simulink model "five_bots_Observer_Obstacle_1_sin_cir"  (R2019b)
settings: Solver=ode5  StartTime=0.0  StopTime=35.0  FixedStep=0.005  RelTol=1e-3
(part 3 of 3)

== matlab function five_bots_Observer_Obstacle_1_sin_cir/Self Calculation 3/APF & Reference Correction/Subsystem/Abstract ==
  data: reference input; agent_x_d output; agent_dot_x_d output; agent_ddot_x_d output
function [agent_x_d, agent_dot_x_d, agent_ddot_x_d] = abstract(reference)

% This function will pick out the reference for the current agent

%% basic parameters
num_agent = 5;
serial_num = 3;
dimension = 3;

% abstract the reference position
x_d = reference (dimension*num_agent*0+1:dimension*num_agent*1);
dot_x_d = reference (dimension*num_agent*1+1:dimension*num_agent*2);
ddot_x_d = reference (dimension*num_agent*2+1:dimension*num_agent*3);

% get the reference for the current agent
agent_x_d = x_d (dimension*(serial_num-1)+1 : dimension*serial_num);
agent_dot_x_d = dot_x_d (dimension*(serial_num-1)+1 : dimension*serial_num);
agent_ddot_x_d = ddot_x_d (dimension*(serial_num-1)+1 : dimension*serial_num);

end

== matlab function five_bots_Observer_Obstacle_1_sin_cir/Self Calculation 3/APF & Reference Correction/Subsystem/Error calculation ==
  data: agent_x_d input; agent_dot_x_d input; pos input; delta_x output; vel input; delta_v output
function [delta_x, delta_v] = error_calculation(agent_x_d, agent_dot_x_d, pos, vel)

delta_x = pos - agent_x_d;
delta_v = vel - agent_dot_x_d;

end

== matlab function five_bots_Observer_Obstacle_1_sin_cir/Self Calculation 3/APF & Reference Correction/Subsystem/Reference Correction ==
  data: agent_x_d input; agent_dot_x_d input; agent_ddot_x_d input; new_x_d output; ob_info input; pos input; vel input; flag_ob input; new_dot_x_d output; new_ddot_x_d output; k_i output
function [new_x_d, new_dot_x_d, new_ddot_x_d,k_i] = fcn(agent_x_d, agent_dot_x_d, agent_ddot_x_d, ob_info, pos, vel, flag_ob)

%% Note
% This function calculates the reference tracking error according to the
% current reference

% input:
% agent_x_d, agent_dot_x_d, agent_ddot_x_d: the given current references
% ob_info: the information of obstacle 
% pos, vel: the current states of agents
% flag_ob: the serial number of the obstacle that the agent might have
% collision with (also the closest one due to one obstacle at a time assumption)

% output:
% new_x_d, new_dot_x_d, new_ddot_x_d: the new references

epsilon_1 = 1.1;

Radius=[0.24;0.23;0.30;0.28;0.25];
serial_num = 1;

dimension = 2; % the dimension of the operating space (x,y)

r_a = Radius(serial_num);
k_i = 0;

if flag_ob ==0 % first if (if the obstacle is far away)
   new_x_d = agent_x_d;
   new_dot_x_d = agent_dot_x_d;
   new_ddot_x_d = agent_ddot_x_d;
else
   %% obtain the obstacle's information
   obstacle = ob_info((dimension+1)*(flag_ob-1)+1 : (dimension+1)*flag_ob); 
   ob_pos = obstacle(1 : dimension);
   agent_pos = pos(1 : dimension);
   r_o = obstacle(dimension+1); 
   %% calculate the distance between the centre of the obstacle and the line generated by current position and reference point
   r_inner = epsilon_1 * (r_a + r_o);
   
   p_o = agent_pos - ob_pos;      % vector between current position and obstacle
   p_d = agent_pos - agent_x_d(1 : dimension);      % vector between current position and reference position
   
   angle = acos(dot(p_o,p_d)/(norm(p_o)*norm(p_d)));    % the angle between the two vectors (rad)
   
   if sin(angle)*norm(p_o) < r_inner && angle < pi/2    % the distance between the p_d line and obstacle is smaller than inner distance and the angle is within 90 degrees
       if sqrt(norm(p_o)^2 - r_inner^2)>norm(p_d) && norm(-p_d+p_o) > r_inner
           new_x_d = agent_x_d;
           new_dot_x_d = agent_dot_x_d;
           new_ddot_x_d = agent_ddot_x_d; 
       else        % here we start to correct the reference
           
           %% find out the two tangents that cross agent's current position
           solu=1;     % number of solutions found
           tan=zeros(2,3);     % parameters of tangent with the form of ax+by+c=0
           k_i = flag_ob;
           
           x1 = agent_pos(1);
           y1 = agent_pos(2);
           
           x2 = ob_pos(1);
           y2 = ob_pos(2);
           
           % find the tangents that are parallel to x/y axis
           if abs(agent_pos(1)-ob_pos(1))==r_inner    % in the form of x=k
               tan(solu,:)=[1,0,-agent_pos(1)];
               solu=solu+1;
           end
           if abs(agent_pos(2)-ob_pos(2))==r_inner
               tan(solu,:)=[0,1,-agent_pos(2)];
               solu=solu+1;
           end
           
           
           if solu==2
               if abs(x1-x2)==r_inner   % in the form of x+ky+b=0
                   a1=(y2-y1)^2-r_inner^2;
                   a2=2*(x2-x1)*(y2-y1);
                   a3=(x2-x1)^2-r_inner^2;
                   k1=(-a2+sqrt(a2^2-4*a1*a3))/(2*a1);
                   k2=(-a2-sqrt(a2^2-4*a1*a3))/(2*a1);
                   if k1==0
                       b=-x1-k2*y1;
                       tan(solu,:)=[1,k2,b];
                   elseif k2==0
                       b=-x1-k1*y1;
                       tan(solu,:)=[1,k1,b];
                   end
               elseif abs(y1-y2)==r_inner   % in the form of kx+y+b=0
                   a1=(x2-x1)^2-r_inner^2;
                   a2=2*(x2-x1)*(y1-y2);
                   a3=(y1-y2)^2-r_inner^2;
                   k1=(-a2+sqrt(a2^2-4*a1*a3))/(2*a1);
                   k2=(-a2-sqrt(a2^2-4*a1*a3))/(2*a1);
                   if k1==0
                       b=-k2*x1-y1;
                       tan(solu,:)=[k2,1,b];
                   elseif k2==0
                       b=-k1*x1-y1;
                       tan(solu,:)=[k1,1,b];
                   end
               end
           elseif solu==1       % no parallel tangents
               a1=(x2-x1)^2-r_inner^2;
               a2=2*(x2-x1)*(y1-y2);
               a3=(y1-y2)^2-r_inner^2;
               k1=(-a2+sqrt(abs(a2^2-4*a1*a3)))/(2*a1);
               k2=(-a2-sqrt(abs(a2^2-4*a1*a3)))/(2*a1);
               %     k1=(-a2+sqrt(a2^2-4*a1*a3))/(2*a1);
               %     k2=(-a2-sqrt(a2^2-4*a1*a3))/(2*a1);
               %     k1=(-a2+sqrt(complex(a2^2-4*a1*a3)))/(2*a1);
               %     k2=(-a2-sqrt(complex(a2^2-4*a1*a3)))/(2*a1);
               b1=y1-k1*x1;
               b2=y1-k2*x1;
               tan(solu,:)=[k1,-1,b1];
               tan(solu+1,:)=[k2,-1,b2];
           end
           
           %% find the optimal tangent
           
           dis_1=abs(tan(1,1)*agent_x_d(1)+tan(1,2)*agent_x_d(2)+tan(1,3))/sqrt(tan(1,1)^2+tan(1,2)^2);
           dis_2=abs(tan(2,1)*agent_x_d(1)+tan(2,2)*agent_x_d(2)+tan(2,3))/sqrt(tan(2,1)^2+tan(2,2)^2);        % distance from reference point to both tangents
           
           if dis_1>=dis_2
               num=2;
           else
               num=1;
           end
           
           op_tan=tan(num,:);
           if op_tan(1)==0
               new_ref=[agent_x_d(1);-op_tan(3)/op_tan(2)];
           elseif op_tan(2)==0
               new_ref=[-op_tan(3)/op_tan(1);agent_x_d(2)];
           else
               mat=[op_tan(1),op_tan(2);op_tan(2),-op_tan(1)];
               new_ref=mat^(-1)*[-op_tan(3);agent_x_d(1)*op_tan(2)-agent_x_d(2)*op_tan(1)];
           end
           
           new_x_d = [new_ref;agent_x_d(3)];
           
           %% get the speed reference's projection on the tangent
           v_ref = agent_dot_x_d(1:dimension);    % speed reference
           vec = new_ref - pos(1:dimension);    % position-position reference vector
           
           angle_vel = acos(dot(v_ref,vec)/(norm(v_ref)*norm(vec)));
           v_pro = norm(v_ref)*cos(angle_vel)*vec/norm(vec);
           new_dot_x_d = [v_pro; agent_dot_x_d(3)];
           
           %% get the acceleration reference's projection on the tangent
           a_ref = agent_ddot_x_d(1:dimension);
           angle_acc = acos(dot(a_ref,vec)/(norm(a_ref)*norm(vec)));
           
           a_pro = norm(a_ref)*cos(angle_acc)*vec/norm(vec);
           new_ddot_x_d = [a_pro; agent_ddot_x_d(3)];
       end
   else 
      new_x_d = agent_x_d;
      new_dot_x_d = agent_dot_x_d;
      new_ddot_x_d = agent_ddot_x_d;          
   end
   
  
       
       
end







end

== matlab function five_bots_Observer_Obstacle_1_sin_cir/Self Calculation 3/MATLAB Function2 ==
  data: x output; delta_x input; y output; theta output
function [x,y,theta] = abs_delta(delta_x)

x = abs(delta_x(1));
y = abs(delta_x(2));
theta = abs(delta_x(3)); 

end

== matlab function five_bots_Observer_Obstacle_1_sin_cir/Self Calculation 3/Observation and selection/Control input transfer ==
  data: u input; u_norm output; pos input
function u_norm = transfer(u, pos)

%% current information
Mass=[4.8;4.5;5.5;5.3;5.0];
Radius=[0.24;0.23;0.30;0.28;0.25];
Inertia=[0.15;0.12;0.25;0.21;0.15];

serial_num = 3; 
dimension = 3;

%% selection
m=Mass(serial_num);
% alpha=Alpha(serial_num);
R=Radius(serial_num);
inertia=Inertia(serial_num);

theta=pos(dimension);

%% calculate g
M=diag([1/m,1/m,1/inertia]);
T=[-sin(theta), -sin(pi/3-theta), sin(pi/3+theta);
    cos(theta), -cos(pi/3-theta), -cos(pi/3+theta);
    R,          R,                  R];

g=M * T;

u_norm = g * u;


end

== matlab function five_bots_Observer_Obstacle_1_sin_cir/Self Calculation 3/Observation and selection/Observer/Observer ==
  data: pos input; vel input; u_norm input; first_hat_dot output; first_hat input; second_hat input; second_hat_dot output
function [first_hat_dot, second_hat_dot] = observer(pos, vel, u_norm, first_hat, second_hat)

% first_hat = [pos_hat; d_hat];         first order states
% second_hat = [vel_hat; w_hat];        second order states

%% parameters

alpha_d1 = 4;
alpha_d2 = 8;
alpha_d3 = 4;

alpha_w1 = 6;
alpha_w2 = 12;
alpha_w3 = 6; 


beta_d = 0.7;
beta_w = 15;

dimension=3;

gamma_d1 = first_hat(dimension*0+1:dimension*1);
gamma_d2 = first_hat(dimension*1+1:dimension*2);
gamma_d3 = first_hat(dimension*2+1:dimension*3);

gamma_w1 = second_hat(dimension*0+1:dimension*1);
gamma_w2 = second_hat(dimension*1+1:dimension*2);
gamma_w3 = second_hat(dimension*2+1:dimension*3);




%% tunning
mu_d1 = -alpha_d1 * power(beta_d,1/3) * power(abs(gamma_d1-pos),2/3) .* sign(gamma_d1-pos) + gamma_d2;
mu_d2 = -alpha_d2 * power(beta_d,1/2) * power(abs(gamma_d2-mu_d1),1/2) .* sign(gamma_d2-mu_d1) + gamma_d3;
mu_d3 = -alpha_d3 * beta_d .* sign(gamma_d3-mu_d2);

mu_w1 = -alpha_w1 * power(beta_w,1/3) * power(abs(gamma_w1-vel),2/3) .* sign(gamma_w1-vel) + gamma_w2;
mu_w2 = -alpha_w2 * power(beta_w,1/2) * power(abs(gamma_w2-mu_w1),1/2) .* sign(gamma_w2-mu_w1) + gamma_w3;
mu_w3 = -alpha_w3 * beta_w .* sign(gamma_w3-mu_w2);



first_hat_dot = [mu_d1 + vel; mu_d2; mu_d3];
second_hat_dot = [mu_w1 + u_norm; mu_w2; mu_w3]; 





end

== matlab function five_bots_Observer_Obstacle_1_sin_cir/Self Calculation 3/Observation and selection/Selecting Information ==
  data: first_hat input; ob_estimation output; second_hat input; first_hat_dot input; d_hat output
function [ob_estimation, d_hat]  = selecting(first_hat, second_hat, first_hat_dot)

dimension=3;

d_hat = first_hat(dimension*1+1 :dimension*2);
w_hat = second_hat(dimension*1+1 : dimension*2);

d_hat_dot = first_hat_dot(dimension*1+1 : dimension*2);

ob_estimation = [d_hat ; w_hat ; d_hat_dot];

end

== matlab function five_bots_Observer_Obstacle_1_sin_cir/Controller and Plant 4/Absolute error ==
  data: x output; e_x input; y output; theta output
function [x,y,theta] = abs_e(e_x)

x = abs(e_x(1));
y = abs(e_x(2));
theta = abs(e_x(3)); 

end

== matlab function five_bots_Observer_Obstacle_1_sin_cir/Controller and Plant 4/MATLAB Function ==
  data: info_commu input; e_xi output; Laplacian input; e_vi output; e_di output
function [e_xi, e_vi, e_di] = commu_sele(info_commu, Laplacian)

%% Note

% The purpose of this function is to 
% 1) abstract the information for calculation
% 2) calculate local variables e_xi, e_vi, e_di

% The info_commu comes in the form of [delta_x; d_hat; delta_v];

%% basic parameters
num_agent = size(Laplacian,1); 
dimension = 3;
serial_num = 4;


%% abstract information from communication
abstract_x = kron(kron(eye(num_agent),[1,0,0]),eye(dimension));
abstract_d = kron(kron(eye(num_agent),[0,1,0]),eye(dimension));
abstract_v = kron(kron(eye(num_agent),[0,0,1]),eye(dimension));

delta_x = abstract_x * info_commu;
d_hat = abstract_d * info_commu;
delta_v = abstract_v * info_commu;

L = Laplacian(serial_num,:);

e_xi = kron(L, eye(dimension) ) * delta_x;
e_di = kron(L, eye(dimension) ) * d_hat;
e_vi = kron(L, eye(dimension) ) * delta_v;







end

== matlab function five_bots_Observer_Obstacle_1_sin_cir/Controller and Plant 4/MATLAB Function1 ==
  data: d input; w input; e_d output; ob_estimation input; e_w output
function [e_d, e_w] = estimation_error(d, w, ob_estimation)

dimension=3;

d_hat = ob_estimation(dimension*0+1 :dimension*1);
w_hat = ob_estimation(dimension*1+1 : dimension*2);


e_d = d_hat - d;
e_w = w_hat - w;

end

== matlab function five_bots_Observer_Obstacle_1_sin_cir/Controller and Plant 4/Mismatched uncertainty/Mismatched disturbance ==
  data: t input; d output
function d = mismatched_disturbance(t)

serial_num=4;
d = [0.3*sin(t+pi*serial_num/5)+0.2; 0.1*cos(1.5*t+pi*serial_num/4)+0.2; 0.2*sin(1.2*t+pi*serial_num/3)+0.1];

end

== matlab function five_bots_Observer_Obstacle_1_sin_cir/Controller and Plant 4/SMC Controller ==
  data: pos input; f_ik input; u output; ddot_x_d input; delta_x input; delta_v input; e_xi input; e_vi input; e_di input; ob_estimation input; s output
function [u,s] = controller(pos, f_ik, ddot_x_d, delta_x, delta_v, e_xi, e_vi, e_di, ob_estimation)

%% Note
% The function for the SMC controller 


%% basic data
Mass=[4.8;4.5;5.5;5.3;5.0];
Radius=[0.24;0.23;0.30;0.28;0.25];
Inertia=[0.15;0.12;0.25;0.21;0.15];

serial_num = 4;
dimension = 3; 

m=Mass(serial_num);
R=Radius(serial_num);
inertia=Inertia(serial_num);


%% observer estimation
d_hat = ob_estimation(dimension*0+1 :dimension*1);
w_hat = ob_estimation(dimension*1+1 : dimension*2);
d_hat_dot = ob_estimation(dimension*2+1 : dimension*3);

%% parameters
lambda = 2;
c = 2;

s = e_vi + e_di + lambda* e_xi;

F = [f_ik ; 0];

%% calculate g_bar
theta = pos(dimension);
M=diag([m,m,inertia]);
T=[-sin(theta), -sin(pi/3-theta), sin(pi/3+theta);
    cos(theta), -cos(pi/3-theta), -cos(pi/3+theta);
    R,          R,                  R];

g_bar = T^-1 * M;

u = g_bar * (-w_hat + ddot_x_d - d_hat_dot - lambda* d_hat - c*s - lambda* delta_v + F - delta_x);

% u = -w_hat + ddot_x_d - d_hat_dot - lambda* d_hat - c*s - lambda* delta_v + F - delta_x;

end

== matlab function five_bots_Observer_Obstacle_1_sin_cir/Controller and Plant 4/System Plant ==
  data: agent_x input; v_dot output; agent_v input; t input; control_input input; w output
function [v_dot, w] = physical_model( agent_x , agent_v, t, control_input )

%% Note
% System output
% v_dot: the acceleration vector
% w: the matched disturbances
% saturation status: off
% model is established by the driving force provided by the motor

%% basic parameters set of agents
Mass=[4.8;4.5;5.5;5.3;5.0];
Radius=[0.24;0.23;0.30;0.28;0.25];
Inertia=[0.15;0.12;0.25;0.21;0.15];

%% assign the parameter according to serial number
serial_num = 4; 
m=Mass(serial_num);
R=Radius(serial_num);
inertia=Inertia(serial_num);

%% current states of the robot
dimension=3;

x=agent_x(1);
y=agent_x(2);
theta=agent_x(dimension);

%% time-varying matched disturbances
% matched_disturbance= [0.5*sin(1.5*t+pi/4*serial_num+x)+2; 0.6*cos(2*t+pi/3*serial_num+0.5*y)+1.5; 0.5*sin(0.8*t+pi/5*serial_num+0.4*theta)+1];

matched_disturbance= [0.5*sin(1.5*t+pi/4*serial_num)+2; 0.6*cos(2*t+pi/3*serial_num)+1.5; 0.5*sin(0.8*t+pi/5*serial_num)+1];

%% the real model of robot
M=diag([1/m,1/m,1/inertia]);
T=[-sin(theta), -sin(pi/3-theta), sin(pi/3+theta);
    cos(theta), -cos(pi/3-theta), -cos(pi/3+theta);
    R,          R,                  R];

% fx = -beta*M*(T*T')*agent_v;


g=M*T;

%% saturation is added here for convinience
% Vmax=6; % the maximum voltage of the motor
% 
% u1up=Vmax/(alpha*m)*(abs(sin(theta))+abs(sin(pi/3-theta))+abs(sin(pi/3+theta)));
% u1do=-Vmax/(alpha*m)*(abs(sin(theta))+abs(sin(pi/3-theta))+abs(sin(pi/3+theta)));
% u2up=Vmax/(alpha*m)*(abs(cos(theta))+abs(cos(pi/3-theta))+abs(cos(pi/3+theta)));
% u2do=-Vmax/(alpha*m)*(abs(cos(theta))+abs(cos(pi/3-theta))+abs(cos(pi/3+theta)));
% u3up=R/(alpha*inertia)*3*Vmax;
% u3do=-R/(alpha*inertia)*3*Vmax;
% 
% control_input(1) = max( min(control_input(1),u1up), u1do );
% control_input(2) = max( min(control_input(2),u2up), u2do );
% control_input(3) = max( min(control_input(3),u3up), u3do );

%% plant output

% w=fx + matched_disturbance; 
w = matched_disturbance;

v_dot = w + g* control_input;


end

== matlab function five_bots_Observer_Obstacle_1_sin_cir/Self Calculation 4/APF & Reference Correction/Find closest obstacle ==
  data: ob_info input; flag_ob output; pos input; f_ik output
function [flag_ob, f_ik] = find_ob(ob_info, pos)

%% Note
% This function will calculate the closest obstacle and see if the agent is
% inside the outer boundaries of the obstacle

% Input:
% ob_info: the information of obstacles
% pos: the position of agents

% Output:
% flag_ob: 0 for outside the boundaries
        %  1 - k for the serial of the obstacle

%% parameters

dimension = 2; % the dimension of the space

epsilon_1 = 1.1; % the parameter for the inner boundaries
epsilon_2 = 2; % the parameter for the outer boundaries

alpha = 2;


Radius=[0.24;0.23;0.30;0.28;0.25];
serial_num = 4;
r_a = Radius(serial_num);

%% find the closest obstacle
flag_ob = 0;
pos_a = pos(1:dimension);
f_ik = [0;0];

for i = 1 : size(ob_info,1)/(dimension+1)
   pos_o = ob_info((dimension+1)*(i-1)+1 : (dimension+1)*(i-1)+dimension);
   r_o = ob_info(i*(dimension+1));
   
   z_ik = pos_a - pos_o;
   
   r_in = epsilon_1 * (r_a + r_o);
   r_out = epsilon_2 * (r_a + r_o);
   
   if norm(z_ik) < epsilon_2 * (r_a + r_o)
       flag_ob = i;
       f_ik = 2* (r_out - norm(z_ik))/(norm(z_ik) - r_in)^2 * z_ik/norm(z_ik);
       break;
   end
    
end




end

== matlab function five_bots_Observer_Obstacle_1_sin_cir/Self Calculation 4/APF & Reference Correction/Subsystem/Abstract ==
  data: reference input; agent_x_d output; agent_dot_x_d output; agent_ddot_x_d output
function [agent_x_d, agent_dot_x_d, agent_ddot_x_d] = abstract(reference)

% This function will pick out the reference for the current agent

%% basic parameters
num_agent = 5;
serial_num = 4;
dimension = 3;

% abstract the reference position
x_d = reference (dimension*num_agent*0+1:dimension*num_agent*1);
dot_x_d = reference (dimension*num_agent*1+1:dimension*num_agent*2);
ddot_x_d = reference (dimension*num_agent*2+1:dimension*num_agent*3);

% get the reference for the current agent
agent_x_d = x_d (dimension*(serial_num-1)+1 : dimension*serial_num);
agent_dot_x_d = dot_x_d (dimension*(serial_num-1)+1 : dimension*serial_num);
agent_ddot_x_d = ddot_x_d (dimension*(serial_num-1)+1 : dimension*serial_num);

end

== matlab function five_bots_Observer_Obstacle_1_sin_cir/Self Calculation 4/APF & Reference Correction/Subsystem/Error calculation ==
  data: agent_x_d input; agent_dot_x_d input; pos input; delta_x output; vel input; delta_v output
function [delta_x, delta_v] = error_calculation(agent_x_d, agent_dot_x_d, pos, vel)

delta_x = pos - agent_x_d;
delta_v = vel - agent_dot_x_d;

end

== matlab function five_bots_Observer_Obstacle_1_sin_cir/Self Calculation 4/APF & Reference Correction/Subsystem/Reference Correction ==
  data: agent_x_d input; agent_dot_x_d input; agent_ddot_x_d input; new_x_d output; ob_info input; pos input; vel input; flag_ob input; new_dot_x_d output; new_ddot_x_d output; k_i output
function [new_x_d, new_dot_x_d, new_ddot_x_d, k_i] = fcn(agent_x_d, agent_dot_x_d, agent_ddot_x_d, ob_info, pos, vel, flag_ob)

%% Note
% This function calculates the reference tracking error according to the
% current reference

% input:
% agent_x_d, agent_dot_x_d, agent_ddot_x_d: the given current references
% ob_info: the information of obstacle 
% pos, vel: the current states of agents
% flag_ob: the serial number of the obstacle that the agent might have
% collision with (also the closest one due to one obstacle at a time assumption)

% output:
% new_x_d, new_dot_x_d, new_ddot_x_d: the new references

epsilon_1 = 1.1;

Radius=[0.24;0.23;0.30;0.28;0.25];
serial_num = 4;

dimension = 2; % the dimension of the operating space (x,y)

r_a = Radius(serial_num);
k_i = 0;

if flag_ob ==0 % first if (if the obstacle is far away)
   new_x_d = agent_x_d;
   new_dot_x_d = agent_dot_x_d;
   new_ddot_x_d = agent_ddot_x_d;
else
   %% obtain the obstacle's information
   obstacle = ob_info((dimension+1)*(flag_ob-1)+1 : (dimension+1)*flag_ob); 
   ob_pos = obstacle(1 : dimension);
   agent_pos = pos(1 : dimension);
   r_o = obstacle(dimension+1); 
   %% calculate the distance between the centre of the obstacle and the line generated by current position and reference point
   r_inner = epsilon_1 * (r_a + r_o);
   
   p_o = agent_pos - ob_pos;      % vector between current position and obstacle
   p_d = agent_pos - agent_x_d(1 : dimension);      % vector between current position and reference position
   
   angle = acos(dot(p_o,p_d)/(norm(p_o)*norm(p_d)));    % the angle between the two vectors (rad)
   
   if sin(angle)*norm(p_o) < r_inner && angle < pi/2    % the distance between the p_d line and obstacle is smaller than inner distance and the angle is within 90 degrees
       if sqrt(norm(p_o)^2 - r_inner^2)>norm(p_d) && norm(-p_d+p_o) > r_inner
           new_x_d = agent_x_d;
           new_dot_x_d = agent_dot_x_d;
           new_ddot_x_d = agent_ddot_x_d; 
       else        % here we start to correct the reference
           
           %% find out the two tangents that cross agent's current position
           solu=1;     % number of solutions found
           tan=zeros(2,3);     % parameters of tangent with the form of ax+by+c=0
           k_i=flag_ob;
           
           x1 = agent_pos(1);
           y1 = agent_pos(2);
           
           x2 = ob_pos(1);
           y2 = ob_pos(2);
           
           % find the tangents that are parallel to x/y axis
           if abs(agent_pos(1)-ob_pos(1))==r_inner    % in the form of x=k
               tan(solu,:)=[1,0,-agent_pos(1)];
               solu=solu+1;
           end
           if abs(agent_pos(2)-ob_pos(2))==r_inner
               tan(solu,:)=[0,1,-agent_pos(2)];
               solu=solu+1;
           end
           
           
           if solu==2
               if abs(x1-x2)==r_inner   % in the form of x+ky+b=0
                   a1=(y2-y1)^2-r_inner^2;
                   a2=2*(x2-x1)*(y2-y1);
                   a3=(x2-x1)^2-r_inner^2;
                   k1=(-a2+sqrt(a2^2-4*a1*a3))/(2*a1);
                   k2=(-a2-sqrt(a2^2-4*a1*a3))/(2*a1);
                   if k1==0
                       b=-x1-k2*y1;
                       tan(solu,:)=[1,k2,b];
                   elseif k2==0
                       b=-x1-k1*y1;
                       tan(solu,:)=[1,k1,b];
                   end
               elseif abs(y1-y2)==r_inner   % in the form of kx+y+b=0
                   a1=(x2-x1)^2-r_inner^2;
                   a2=2*(x2-x1)*(y1-y2);
                   a3=(y1-y2)^2-r_inner^2;
                   k1=(-a2+sqrt(a2^2-4*a1*a3))/(2*a1);
                   k2=(-a2-sqrt(a2^2-4*a1*a3))/(2*a1);
                   if k1==0
                       b=-k2*x1-y1;
                       tan(solu,:)=[k2,1,b];
                   elseif k2==0
                       b=-k1*x1-y1;
                       tan(solu,:)=[k1,1,b];
                   end
               end
           elseif solu==1       % no parallel tangents
               a1=(x2-x1)^2-r_inner^2;
               a2=2*(x2-x1)*(y1-y2);
               a3=(y1-y2)^2-r_inner^2;
               k1=(-a2+sqrt(abs(a2^2-4*a1*a3)))/(2*a1);
               k2=(-a2-sqrt(abs(a2^2-4*a1*a3)))/(2*a1);
               %     k1=(-a2+sqrt(a2^2-4*a1*a3))/(2*a1);
               %     k2=(-a2-sqrt(a2^2-4*a1*a3))/(2*a1);
               %     k1=(-a2+sqrt(complex(a2^2-4*a1*a3)))/(2*a1);
               %     k2=(-a2-sqrt(complex(a2^2-4*a1*a3)))/(2*a1);
               b1=y1-k1*x1;
               b2=y1-k2*x1;
               tan(solu,:)=[k1,-1,b1];
               tan(solu+1,:)=[k2,-1,b2];
           end
           
           %% find the optimal tangent
           
           dis_1=abs(tan(1,1)*agent_x_d(1)+tan(1,2)*agent_x_d(2)+tan(1,3))/sqrt(tan(1,1)^2+tan(1,2)^2);
           dis_2=abs(tan(2,1)*agent_x_d(1)+tan(2,2)*agent_x_d(2)+tan(2,3))/sqrt(tan(2,1)^2+tan(2,2)^2);        % distance from reference point to both tangents
           
           if dis_1>=dis_2
               num=2;
           else
               num=1;
           end
           
           op_tan=tan(num,:);
           if op_tan(1)==0
               new_ref=[agent_x_d(1);-op_tan(3)/op_tan(2)];
           elseif op_tan(2)==0
               new_ref=[-op_tan(3)/op_tan(1);agent_x_d(2)];
           else
               mat=[op_tan(1),op_tan(2);op_tan(2),-op_tan(1)];
               new_ref=mat^(-1)*[-op_tan(3);agent_x_d(1)*op_tan(2)-agent_x_d(2)*op_tan(1)];
           end
           
           new_x_d = [new_ref;agent_x_d(3)];
           
           %% get the speed reference's projection on the tangent
           v_ref = agent_dot_x_d(1:dimension);    % speed reference
           vec = new_ref - pos(1:dimension);    % position-position reference vector
           
           angle_vel = acos(dot(v_ref,vec)/(norm(v_ref)*norm(vec)));
           v_pro = norm(v_ref)*cos(angle_vel)*vec/norm(vec);
           new_dot_x_d = [v_pro; agent_dot_x_d(3)];
           
           %% get the acceleration reference's projection on the tangent
           a_ref = agent_ddot_x_d(1:dimension);
           angle_acc = acos(dot(a_ref,vec)/(norm(a_ref)*norm(vec)));
           
           a_pro = norm(a_ref)*cos(angle_acc)*vec/norm(vec);
           new_ddot_x_d = [a_pro; agent_ddot_x_d(3)];
       end
   else 
      new_x_d = agent_x_d;
      new_dot_x_d = agent_dot_x_d;
      new_ddot_x_d = agent_ddot_x_d;          
   end
   
  
       
       
end







end

== matlab function five_bots_Observer_Obstacle_1_sin_cir/Self Calculation 4/MATLAB Function2 ==
  data: x output; delta_x input; y output; theta output
function [x,y,theta] = abs_delta(delta_x)

x = abs(delta_x(1));
y = abs(delta_x(2));
theta = abs(delta_x(3)); 

end

== matlab function five_bots_Observer_Obstacle_1_sin_cir/Self Calculation 4/Observation and selection/Control input transfer ==
  data: u input; u_norm output; pos input
function u_norm = transfer(u, pos)

%% current information
Mass=[4.8;4.5;5.5;5.3;5.0];
Radius=[0.24;0.23;0.30;0.28;0.25];
Inertia=[0.15;0.12;0.25;0.21;0.15];

serial_num = 4; 
dimension = 3;

%% selection
m=Mass(serial_num);
R=Radius(serial_num);
inertia=Inertia(serial_num);

theta=pos(dimension);

%% calculate g
M=diag([1/m,1/m,1/inertia]);
T=[-sin(theta), -sin(pi/3-theta), sin(pi/3+theta);
    cos(theta), -cos(pi/3-theta), -cos(pi/3+theta);
    R,          R,                  R];

g=M * T;

u_norm = g * u;


end

== matlab function five_bots_Observer_Obstacle_1_sin_cir/Self Calculation 4/Observation and selection/Observer/Observer ==
  data: pos input; vel input; u_norm input; first_hat_dot output; first_hat input; second_hat input; second_hat_dot output
function [first_hat_dot, second_hat_dot] = observer(pos, vel, u_norm, first_hat, second_hat)

% first_hat = [pos_hat; d_hat];         first order states
% second_hat = [vel_hat; w_hat];        second order states

%% parameters

alpha_d1 = 4;
alpha_d2 = 8;
alpha_d3 = 4;

alpha_w1 = 6;
alpha_w2 = 12;
alpha_w3 = 6; 


beta_d = 0.7;
beta_w = 15;

dimension=3;

gamma_d1 = first_hat(dimension*0+1:dimension*1);
gamma_d2 = first_hat(dimension*1+1:dimension*2);
gamma_d3 = first_hat(dimension*2+1:dimension*3);

gamma_w1 = second_hat(dimension*0+1:dimension*1);
gamma_w2 = second_hat(dimension*1+1:dimension*2);
gamma_w3 = second_hat(dimension*2+1:dimension*3);




%% tunning
mu_d1 = -alpha_d1 * power(beta_d,1/3) * power(abs(gamma_d1-pos),2/3) .* sign(gamma_d1-pos) + gamma_d2;
mu_d2 = -alpha_d2 * power(beta_d,1/2) * power(abs(gamma_d2-mu_d1),1/2) .* sign(gamma_d2-mu_d1) + gamma_d3;
mu_d3 = -alpha_d3 * beta_d .* sign(gamma_d3-mu_d2);

mu_w1 = -alpha_w1 * power(beta_w,1/3) * power(abs(gamma_w1-vel),2/3) .* sign(gamma_w1-vel) + gamma_w2;
mu_w2 = -alpha_w2 * power(beta_w,1/2) * power(abs(gamma_w2-mu_w1),1/2) .* sign(gamma_w2-mu_w1) + gamma_w3;
mu_w3 = -alpha_w3 * beta_w .* sign(gamma_w3-mu_w2);



first_hat_dot = [mu_d1 + vel; mu_d2; mu_d3];
second_hat_dot = [mu_w1 + u_norm; mu_w2; mu_w3]; 





end

== matlab function five_bots_Observer_Obstacle_1_sin_cir/Self Calculation 4/Observation and selection/Selecting Information ==
  data: first_hat input; ob_estimation output; second_hat input; first_hat_dot input; d_hat output
function [ob_estimation, d_hat]  = selecting(first_hat, second_hat, first_hat_dot)

dimension=3;

d_hat = first_hat(dimension*1+1 :dimension*2);
w_hat = second_hat(dimension*1+1 : dimension*2);

d_hat_dot = first_hat_dot(dimension*1+1 : dimension*2);

ob_estimation = [d_hat ; w_hat ; d_hat_dot];

end

== matlab function five_bots_Observer_Obstacle_1_sin_cir/Controller and Plant 5/Absolute error ==
  data: x output; e_x input; y output; theta output
function [x,y,theta] = abs_e(e_x)

x = abs(e_x(1));
y = abs(e_x(2));
theta = abs(e_x(3)); 

end

== matlab function five_bots_Observer_Obstacle_1_sin_cir/Controller and Plant 5/MATLAB Function ==
  data: info_commu input; e_xi output; Laplacian input; e_vi output; e_di output
function [e_xi, e_vi, e_di] = commu_sele(info_commu, Laplacian)

%% Note

% The purpose of this function is to 
% 1) abstract the information for calculation
% 2) calculate local variables e_xi, e_vi, e_di

% The info_commu comes in the form of [delta_x; d_hat; delta_v];

%% basic parameters
num_agent = size(Laplacian,1); 
dimension = 3;
serial_num = 5;


%% abstract information from communication
abstract_x = kron(kron(eye(num_agent),[1,0,0]),eye(dimension));
abstract_d = kron(kron(eye(num_agent),[0,1,0]),eye(dimension));
abstract_v = kron(kron(eye(num_agent),[0,0,1]),eye(dimension));

delta_x = abstract_x * info_commu;
d_hat = abstract_d * info_commu;
delta_v = abstract_v * info_commu;

L = Laplacian(serial_num,:);

e_xi = kron(L, eye(dimension) ) * delta_x;
e_di = kron(L, eye(dimension) ) * d_hat;
e_vi = kron(L, eye(dimension) ) * delta_v;







end

== matlab function five_bots_Observer_Obstacle_1_sin_cir/Controller and Plant 5/MATLAB Function1 ==
  data: d input; w input; e_d output; ob_estimation input; e_w output
function [e_d, e_w] = estimation_error(d, w, ob_estimation)

dimension=3;

d_hat = ob_estimation(dimension*0+1 :dimension*1);
w_hat = ob_estimation(dimension*1+1 : dimension*2);


e_d = d_hat - d;
e_w = w_hat - w;

end

== matlab function five_bots_Observer_Obstacle_1_sin_cir/Controller and Plant 5/Mismatched uncertainty/Mismatched disturbance ==
  data: t input; d output
function d = mismatched_disturbance(t)

serial_num=5;
d = [0.3*sin(t+pi*serial_num/5)+0.2; 0.1*cos(1.5*t+pi*serial_num/4)+0.2; 0.2*sin(1.2*t+pi*serial_num/3)+0.1];

end

== matlab function five_bots_Observer_Obstacle_1_sin_cir/Controller and Plant 5/SMC Controller ==
  data: pos input; f_ik input; u output; ddot_x_d input; delta_x input; delta_v input; e_xi input; e_vi input; e_di input; ob_estimation input; s output
function [u,s] = controller(pos, f_ik, ddot_x_d, delta_x, delta_v, e_xi, e_vi, e_di, ob_estimation)

%% Note
% The function for the SMC controller 


%% basic data
Mass=[4.8;4.5;5.5;5.3;5.0];
Radius=[0.24;0.23;0.30;0.28;0.25];
Inertia=[0.15;0.12;0.25;0.21;0.15];

serial_num = 5;
dimension = 3; 

m=Mass(serial_num);
R=Radius(serial_num);
inertia=Inertia(serial_num);


%% observer estimation
d_hat = ob_estimation(dimension*0+1 :dimension*1);
w_hat = ob_estimation(dimension*1+1 : dimension*2);
d_hat_dot = ob_estimation(dimension*2+1 : dimension*3);

%% parameters
lambda = 2;
c = 2;

s = e_vi + e_di + lambda* e_xi;

F = [f_ik ; 0];

%% calculate g_bar
theta = pos(dimension);
M=diag([m,m,inertia]);
T=[-sin(theta), -sin(pi/3-theta), sin(pi/3+theta);
    cos(theta), -cos(pi/3-theta), -cos(pi/3+theta);
    R,          R,                  R];

g_bar = T^-1 * M;

u = g_bar * (-w_hat + ddot_x_d - d_hat_dot - lambda* d_hat - c*s - lambda* delta_v + F - delta_x);

% u = -w_hat + ddot_x_d - d_hat_dot - lambda* d_hat - c*s - lambda* delta_v + F - delta_x;

end

== matlab function five_bots_Observer_Obstacle_1_sin_cir/Controller and Plant 5/System Plant ==
  data: agent_x input; v_dot output; agent_v input; t input; control_input input; w output
function [v_dot, w] = physical_model( agent_x , agent_v, t, control_input )

%% Note
% System output
% v_dot: the acceleration vector
% w: the matched disturbances
% saturation status: off
% model is established by the driving force provided by the motor

%% basic parameters set of agents
Mass=[4.8;4.5;5.5;5.3;5.0];
Radius=[0.24;0.23;0.30;0.28;0.25];
Inertia=[0.15;0.12;0.25;0.21;0.15];

%% assign the parameter according to serial number
serial_num = 5; 
m=Mass(serial_num);
% alpha=Alpha(serial_num);
R=Radius(serial_num);
inertia=Inertia(serial_num);
% beta=Beta(serial_num);

%% current states of the robot
dimension=3;

x=agent_x(1);
y=agent_x(2);
theta=agent_x(dimension);

%% time-varying matched disturbances
% matched_disturbance= [0.5*sin(1.5*t+pi/4*serial_num+x)+2; 0.6*cos(2*t+pi/3*serial_num+0.5*y)+1.5; 0.5*sin(0.8*t+pi/5*serial_num+0.4*theta)+1];

matched_disturbance= [0.5*sin(1.5*t+pi/4*serial_num)+2; 0.6*cos(2*t+pi/3*serial_num)+1.5; 0.5*sin(0.8*t+pi/5*serial_num)+1];

%% the real model of robot
M=diag([1/m,1/m,1/inertia]);
T=[-sin(theta), -sin(pi/3-theta), sin(pi/3+theta);
    cos(theta), -cos(pi/3-theta), -cos(pi/3+theta);
    R,          R,                  R];

% fx = -beta*M*(T*T')*agent_v;


g=M*T;

%% saturation is added here for convinience
% Vmax=6; % the maximum voltage of the motor
% 
% u1up=Vmax/(alpha*m)*(abs(sin(theta))+abs(sin(pi/3-theta))+abs(sin(pi/3+theta)));
% u1do=-Vmax/(alpha*m)*(abs(sin(theta))+abs(sin(pi/3-theta))+abs(sin(pi/3+theta)));
% u2up=Vmax/(alpha*m)*(abs(cos(theta))+abs(cos(pi/3-theta))+abs(cos(pi/3+theta)));
% u2do=-Vmax/(alpha*m)*(abs(cos(theta))+abs(cos(pi/3-theta))+abs(cos(pi/3+theta)));
% u3up=R/(alpha*inertia)*3*Vmax;
% u3do=-R/(alpha*inertia)*3*Vmax;
% 
% control_input(1) = max( min(control_input(1),u1up), u1do );
% control_input(2) = max( min(control_input(2),u2up), u2do );
% control_input(3) = max( min(control_input(3),u3up), u3do );

%% plant output

% w=fx + matched_disturbance; 
w = matched_disturbance;

v_dot = w + g* control_input;


end

== matlab function five_bots_Observer_Obstacle_1_sin_cir/Self Calculation 5/APF & Reference Correction/Find closest obstacle ==
  data: ob_info input; flag_ob output; pos input; f_ik output
function [flag_ob, f_ik] = find_ob(ob_info, pos)

%% Note
% This function will calculate the closest obstacle and see if the agent is
% inside the outer boundaries of the obstacle

% Input:
% ob_info: the information of obstacles
% pos: the position of agents

% Output:
% flag_ob: 0 for outside the boundaries
        %  1 - k for the serial of the obstacle

%% parameters

dimension = 2; % the dimension of the space

epsilon_1 = 1.1; % the parameter for the inner boundaries
epsilon_2 = 2; % the parameter for the outer boundaries

alpha = 2;


Radius=[0.24;0.23;0.30;0.28;0.25];
serial_num = 5;
r_a = Radius(serial_num);

%% find the closest obstacle
flag_ob = 0;
pos_a = pos(1:dimension);
f_ik = [0;0];

for i = 1 : size(ob_info,1)/(dimension+1)
   pos_o = ob_info((dimension+1)*(i-1)+1 : (dimension+1)*(i-1)+dimension);
   r_o = ob_info(i*(dimension+1));
   
   z_ik = pos_a - pos_o;
   
   r_in = epsilon_1 * (r_a + r_o);
   r_out = epsilon_2 * (r_a + r_o);
   
   if norm(z_ik) < epsilon_2 * (r_a + r_o)
       flag_ob = i;
       f_ik = alpha* (r_out - norm(z_ik))/(norm(z_ik) - r_in)^2 * z_ik/norm(z_ik);
       break;
   end
    
end




end

== matlab function five_bots_Observer_Obstacle_1_sin_cir/Self Calculation 5/APF & Reference Correction/Subsystem/Abstract ==
  data: reference input; agent_x_d output; agent_dot_x_d output; agent_ddot_x_d output
function [agent_x_d, agent_dot_x_d, agent_ddot_x_d] = abstract(reference)

% This function will pick out the reference for the current agent

%% basic parameters
num_agent = 5;
serial_num = 5;
dimension = 3;

% abstract the reference position
x_d = reference (dimension*num_agent*0+1:dimension*num_agent*1);
dot_x_d = reference (dimension*num_agent*1+1:dimension*num_agent*2);
ddot_x_d = reference (dimension*num_agent*2+1:dimension*num_agent*3);

% get the reference for the current agent
agent_x_d = x_d (dimension*(serial_num-1)+1 : dimension*serial_num);
agent_dot_x_d = dot_x_d (dimension*(serial_num-1)+1 : dimension*serial_num);
agent_ddot_x_d = ddot_x_d (dimension*(serial_num-1)+1 : dimension*serial_num);

end

== matlab function five_bots_Observer_Obstacle_1_sin_cir/Self Calculation 5/APF & Reference Correction/Subsystem/Error calculation ==
  data: agent_x_d input; agent_dot_x_d input; pos input; delta_x output; vel input; delta_v output
function [delta_x, delta_v] = error_calculation(agent_x_d, agent_dot_x_d, pos, vel)

delta_x = pos - agent_x_d;
delta_v = vel - agent_dot_x_d;

end

== matlab function five_bots_Observer_Obstacle_1_sin_cir/Self Calculation 5/APF & Reference Correction/Subsystem/Reference Correction ==
  data: agent_x_d input; agent_dot_x_d input; agent_ddot_x_d input; new_x_d output; ob_info input; pos input; vel input; flag_ob input; new_dot_x_d output; new_ddot_x_d output; k_i output
function [new_x_d, new_dot_x_d, new_ddot_x_d, k_i] = fcn(agent_x_d, agent_dot_x_d, agent_ddot_x_d, ob_info, pos, vel, flag_ob)

%% Note
% This function calculates the reference tracking error according to the
% current reference

% input:
% agent_x_d, agent_dot_x_d, agent_ddot_x_d: the given current references
% ob_info: the information of obstacle 
% pos, vel: the current states of agents
% flag_ob: the serial number of the obstacle that the agent might have
% collision with (also the closest one due to one obstacle at a time assumption)

% output:
% new_x_d, new_dot_x_d, new_ddot_x_d: the new references

epsilon_1 = 1.1;

Radius=[0.24;0.23;0.30;0.28;0.25];
serial_num = 5;

dimension = 2; % the dimension of the operating space (x,y)

r_a = Radius(serial_num);
k_i = 0;

if flag_ob ==0 % first if (if the obstacle is far away)
   new_x_d = agent_x_d;
   new_dot_x_d = agent_dot_x_d;
   new_ddot_x_d = agent_ddot_x_d;
else
   %% obtain the obstacle's information
   obstacle = ob_info((dimension+1)*(flag_ob-1)+1 : (dimension+1)*flag_ob); 
   ob_pos = obstacle(1 : dimension);
   agent_pos = pos(1 : dimension);
   r_o = obstacle(dimension+1); 
   %% calculate the distance between the centre of the obstacle and the line generated by current position and reference point
   r_inner = epsilon_1 * (r_a + r_o);
   
   p_o = agent_pos - ob_pos;      % vector between current position and obstacle
   p_d = agent_pos - agent_x_d(1 : dimension);      % vector between current position and reference position
   
   angle = acos(dot(p_o,p_d)/(norm(p_o)*norm(p_d)));    % the angle between the two vectors (rad)
   
   if sin(angle)*norm(p_o) < r_inner && angle < pi/2    % the distance between the p_d line and obstacle is smaller than inner distance and the angle is within 90 degrees
       if sqrt(norm(p_o)^2 - r_inner^2)>norm(p_d) && norm(-p_d+p_o) > r_inner
           new_x_d = agent_x_d;
           new_dot_x_d = agent_dot_x_d;
           new_ddot_x_d = agent_ddot_x_d; 
       else        % here we start to correct the reference
           
           %% find out the two tangents that cross agent's current position
           solu=1;     % number of solutions found
           tan=zeros(2,3);     % parameters of tangent with the form of ax+by+c=0
           k_i = flag_ob;
           
           x1 = agent_pos(1);
           y1 = agent_pos(2);
           
           x2 = ob_pos(1);
           y2 = ob_pos(2);
           
           % find the tangents that are parallel to x/y axis
           if abs(agent_pos(1)-ob_pos(1))==r_inner    % in the form of x=k
               tan(solu,:)=[1,0,-agent_pos(1)];
               solu=solu+1;
           end
           if abs(agent_pos(2)-ob_pos(2))==r_inner
               tan(solu,:)=[0,1,-agent_pos(2)];
               solu=solu+1;
           end
           
           
           if solu==2
               if abs(x1-x2)==r_inner   % in the form of x+ky+b=0
                   a1=(y2-y1)^2-r_inner^2;
                   a2=2*(x2-x1)*(y2-y1);
                   a3=(x2-x1)^2-r_inner^2;
                   k1=(-a2+sqrt(a2^2-4*a1*a3))/(2*a1);
                   k2=(-a2-sqrt(a2^2-4*a1*a3))/(2*a1);
                   if k1==0
                       b=-x1-k2*y1;
                       tan(solu,:)=[1,k2,b];
                   elseif k2==0
                       b=-x1-k1*y1;
                       tan(solu,:)=[1,k1,b];
                   end
               elseif abs(y1-y2)==r_inner   % in the form of kx+y+b=0
                   a1=(x2-x1)^2-r_inner^2;
                   a2=2*(x2-x1)*(y1-y2);
                   a3=(y1-y2)^2-r_inner^2;
                   k1=(-a2+sqrt(a2^2-4*a1*a3))/(2*a1);
                   k2=(-a2-sqrt(a2^2-4*a1*a3))/(2*a1);
                   if k1==0
                       b=-k2*x1-y1;
                       tan(solu,:)=[k2,1,b];
                   elseif k2==0
                       b=-k1*x1-y1;
                       tan(solu,:)=[k1,1,b];
                   end
               end
           elseif solu==1       % no parallel tangents
               a1=(x2-x1)^2-r_inner^2;
               a2=2*(x2-x1)*(y1-y2);
               a3=(y1-y2)^2-r_inner^2;
               k1=(-a2+sqrt(abs(a2^2-4*a1*a3)))/(2*a1);
               k2=(-a2-sqrt(abs(a2^2-4*a1*a3)))/(2*a1);
               %     k1=(-a2+sqrt(a2^2-4*a1*a3))/(2*a1);
               %     k2=(-a2-sqrt(a2^2-4*a1*a3))/(2*a1);
               %     k1=(-a2+sqrt(complex(a2^2-4*a1*a3)))/(2*a1);
               %     k2=(-a2-sqrt(complex(a2^2-4*a1*a3)))/(2*a1);
               b1=y1-k1*x1;
               b2=y1-k2*x1;
               tan(solu,:)=[k1,-1,b1];
               tan(solu+1,:)=[k2,-1,b2];
           end
           
           %% find the optimal tangent
           
           dis_1=abs(tan(1,1)*agent_x_d(1)+tan(1,2)*agent_x_d(2)+tan(1,3))/sqrt(tan(1,1)^2+tan(1,2)^2);
           dis_2=abs(tan(2,1)*agent_x_d(1)+tan(2,2)*agent_x_d(2)+tan(2,3))/sqrt(tan(2,1)^2+tan(2,2)^2);        % distance from reference point to both tangents
           
           if dis_1>=dis_2
               num=2;
           else
               num=1;
           end
           
           op_tan=tan(num,:);
           if op_tan(1)==0
               new_ref=[agent_x_d(1);-op_tan(3)/op_tan(2)];
           elseif op_tan(2)==0
               new_ref=[-op_tan(3)/op_tan(1);agent_x_d(2)];
           else
               mat=[op_tan(1),op_tan(2);op_tan(2),-op_tan(1)];
               new_ref=mat^(-1)*[-op_tan(3);agent_x_d(1)*op_tan(2)-agent_x_d(2)*op_tan(1)];
           end
           
           new_x_d = [new_ref;agent_x_d(3)];
           
           %% get the speed reference's projection on the tangent
           v_ref = agent_dot_x_d(1:dimension);    % speed reference
           vec = new_ref - pos(1:dimension);    % position-position reference vector
           
           angle_vel = acos(dot(v_ref,vec)/(norm(v_ref)*norm(vec)));
           v_pro = norm(v_ref)*cos(angle_vel)*vec/norm(vec);
           new_dot_x_d = [v_pro; agent_dot_x_d(3)];
           
           %% get the acceleration reference's projection on the tangent
           a_ref = agent_ddot_x_d(1:dimension);
           angle_acc = acos(dot(a_ref,vec)/(norm(a_ref)*norm(vec)));
           
           a_pro = norm(a_ref)*cos(angle_acc)*vec/norm(vec);
           new_ddot_x_d = [a_pro; agent_ddot_x_d(3)];
       end
   else 
      new_x_d = agent_x_d;
      new_dot_x_d = agent_dot_x_d;
      new_ddot_x_d = agent_ddot_x_d;          
   end
   
  
       
       
end







end

== matlab function five_bots_Observer_Obstacle_1_sin_cir/Self Calculation 5/MATLAB Function2 ==
  data: x output; delta_x input; y output; theta output
function [x,y,theta] = abs_delta(delta_x)

x = abs(delta_x(1));
y = abs(delta_x(2));
theta = abs(delta_x(3)); 

end

== matlab function five_bots_Observer_Obstacle_1_sin_cir/Self Calculation 5/Observation and selection/Control input transfer ==
  data: u input; u_norm output; pos input
function u_norm = transfer(u, pos)

%% current information
Mass=[4.8;4.5;5.5;5.3;5.0];
Radius=[0.24;0.23;0.30;0.28;0.25];
Inertia=[0.15;0.12;0.25;0.21;0.15];

serial_num = 5; 
dimension = 3;

%% selection
m=Mass(serial_num);
R=Radius(serial_num);
inertia=Inertia(serial_num);

theta=pos(dimension);

%% calculate g
M=diag([1/m,1/m,1/inertia]);
T=[-sin(theta), -sin(pi/3-theta), sin(pi/3+theta);
    cos(theta), -cos(pi/3-theta), -cos(pi/3+theta);
    R,          R,                  R];

g=M * T;

u_norm = g * u;


end

== matlab function five_bots_Observer_Obstacle_1_sin_cir/Self Calculation 5/Observation and selection/Observer/Observer ==
  data: pos input; vel input; u_norm input; first_hat_dot output; first_hat input; second_hat input; second_hat_dot output
function [first_hat_dot, second_hat_dot] = observer(pos, vel, u_norm, first_hat, second_hat)

% first_hat = [pos_hat; d_hat];         first order states
% second_hat = [vel_hat; w_hat];        second order states

%% parameters

alpha_d1 = 4;
alpha_d2 = 8;
alpha_d3 = 4;

alpha_w1 = 6;
alpha_w2 = 12;
alpha_w3 = 6; 


beta_d = 0.7;
beta_w = 15;

dimension=3;

gamma_d1 = first_hat(dimension*0+1:dimension*1);
gamma_d2 = first_hat(dimension*1+1:dimension*2);
gamma_d3 = first_hat(dimension*2+1:dimension*3);

gamma_w1 = second_hat(dimension*0+1:dimension*1);
gamma_w2 = second_hat(dimension*1+1:dimension*2);
gamma_w3 = second_hat(dimension*2+1:dimension*3);




%% tunning
mu_d1 = -alpha_d1 * power(beta_d,1/3) * power(abs(gamma_d1-pos),2/3) .* sign(gamma_d1-pos) + gamma_d2;
mu_d2 = -alpha_d2 * power(beta_d,1/2) * power(abs(gamma_d2-mu_d1),1/2) .* sign(gamma_d2-mu_d1) + gamma_d3;
mu_d3 = -alpha_d3 * beta_d .* sign(gamma_d3-mu_d2);

mu_w1 = -alpha_w1 * power(beta_w,1/3) * power(abs(gamma_w1-vel),2/3) .* sign(gamma_w1-vel) + gamma_w2;
mu_w2 = -alpha_w2 * power(beta_w,1/2) * power(abs(gamma_w2-mu_w1),1/2) .* sign(gamma_w2-mu_w1) + gamma_w3;
mu_w3 = -alpha_w3 * beta_w .* sign(gamma_w3-mu_w2);



first_hat_dot = [mu_d1 + vel; mu_d2; mu_d3];
second_hat_dot = [mu_w1 + u_norm; mu_w2; mu_w3]; 





end

== matlab function five_bots_Observer_Obstacle_1_sin_cir/Self Calculation 5/Observation and selection/Selecting Information ==
  data: first_hat input; ob_estimation output; second_hat input; first_hat_dot input; d_hat output
function [ob_estimation, d_hat]  = selecting(first_hat, second_hat, first_hat_dot)

dimension=3;

d_hat = first_hat(dimension*1+1 :dimension*2);
w_hat = second_hat(dimension*1+1 : dimension*2);

d_hat_dot = first_hat_dot(dimension*1+1 : dimension*2);

ob_estimation = [d_hat ; w_hat ; d_hat_dot];

end
